simulink model "edgeDet_try2"  (R2013b)
settings: Solver=ode45  StartTime=0.0  StopTime=10.0  RelTol=1e-3
settings Model: Creator=aidan  LastModifiedBy=aidan

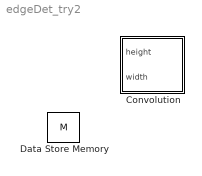
== system edgeDet_try2 ==
  Convolution : Stateflow chart  TreatAsAtomicUnit=on
  Data Store Memory : DataStoreMemory  DataStoreName=M  ReadBeforeWriteMsg=warning  WriteAfterWriteMsg=warning  WriteAfterReadMsg=warning  InitialValue=[0 0 0; 0 0 0; 0 0 0]  OutDataTypeStr=double

== stateflow chart edgeDet_try2/Convolution ==
  state InitialState
    x=0;
    y=0;
  state Select_Matrix
    %A = M[1](x-1:x+1,y-1:y+1);
    %Dont' need this til we parallelize,
    % also not worrying about extra border pixels
  state Operations [group]
    state Inner Loop [group]
      (junction 52) -> (junction 57) [order 1] : [j < 3]
      (junction 57) -> (junction 53) [order 1]
      (junction 53) -> (junction 52) : {j++;}
    (junction 56) -> (junction 51) [order 2] : [i<3]
    (junction 51) -> (junction 52) : {j=0;}
    (junction 55) -> (junction 56) : {i++;}
    (junction 57) -> (junction 53) [order 2] : [j==2&&i==2]
    (junction 52) -> (junction 55) [order 2]
  state WritetoFile
    %Write to the Really big Matrix
    %Value of SUM into location (X,Y) with offset
  state FinalState
  state Do_Math
    %en:
    %Gx = [-1, 0, 1; -2, 0, 2;-1, 0, 1];
    %Gy = [1 2 1;  0 0 0; -1 -2 -1];
    %SUM_X = 0;
    %SUM_Y = 0;
    %for i = 1:3
    % for j = 1:3
    %if(i != 2, j != 2)
    %	SUM_X = SUM_X + Gx(i, j) * A(i,j);
    %	SUM_Y = SUM_Y + Gy(i, j) * A(i,j);
    %end
    % end
    %end
  (default) -> InitialState
  InitialState -> (junction 59) : {x=0;}
  (junction 59) -> (junction 63) [order 1] : [x<height]
  (junction 67) -> (junction 59) [order 2] : {x++;}
  (junction 59) -> FinalState [order 2]
  (junction 63) -> (junction 67) : {y=0;}
  (junction 67) -> (junction 50) [order 1] : [y<width]
  (junction 50) -> (junction 56) : {i=0;}
  WritetoFile -> (junction 67) : {y++;}
  (junction 56) -> WritetoFile [order 1]
  data: x local double; y local double; M data_store_memory; height input; width input; i local double; j local double
